simulink model "newPVmethod_1"  (R2024b)
settings: Solver=FixedStepDiscrete  StartTime=0.0  StopTime=20  FixedStep=1e-6  MaxStep=1e-6  MinStep=1e-6  RelTol=1e-3
values from neighbouring files (symbols this model uses):
  a0_ipv = kp_ipv*(1 + ts/ti_ipv)    (= 0.108333333333)    [PV_sim_init.m]    (also in controller_init.m = 0.0541666666667)
  a0_vpv = kp_vpv*(1 + ts/ti_vpv)    (= 0.100769230769)    [PV_sim_init.m]    (also in controller_init.m)
  a1_ipv = -kp_ipv    (= -0.1)    [PV_sim_init.m]    (also in controller_init.m = -0.05)
  a1_vpv = -kp_vpv    (= -0.1)    [PV_sim_init.m]    (also in controller_init.m)
  Vdc_sim = 400    [PV_sim_init.m]
undefined symbols (not defined in the file or in its folder): sigbuilder_block
libraries: spsSeriesRLCBranchLib x7, slpidlib x6, simulink x5, spsCurrentMeasurementLib x2, spsDCVoltageSourceLib x2, spsPVArrayLib x2, spsVoltageMeasurementLib x2, spsIGBTDiodeLib x2, spsControlledCurrentSourceLib x1, spsControlledVoltageSourceLib x1, spspowerguiLib x1, spsDiodeLib x1
(part 2 of 3)

== matlab function newPVmethod_1/basic_prc_2 ==
  data: Preserve input; c input; Vpv input; Ipv input; Vref output; timer input; D output; out output; reset input
function [Vref,D,out] = RefGen(Preserve,c,Vpv,Ipv,timer,reset)
% main function to execute every time

%variables to remember each execution
persistent state outprev
% global mppt_len measure_len operate_len MPP_SLOPE RESPOW_THRESH REPEAT_THRESH
% global NEW_POINT DEAD_CYCLES MAX_CYCLES

% mppt_len = 1;
% measure_len = 1;
% operate_len = 7;
MAX_CYCLES = 1999;
DEAD_CYCLES = MAX_CYCLES - 1000;
VREF_MAX = 360;
VREF_MIN = 0;
V_BUS_NOMINAL = 400;

%initialize
if isempty(state)
    state = init_state();
    state.Preserve = Preserve;
    outprev = zeros(1,2);
end
out = outprev;
Vref = state.Vrefprev;
dP = 0;
dV = 0;

% if Preserve == 100
%     % for i = 1:1:state.k
%     %     state.Ppva(i) = 0;
%     %     state.Vpva(i) = 0;
%     % end
%     % state.k = 1;
%     state.mode = 0;
%     % state.Preserve = Preserve;
% end

if c>DEAD_CYCLES && c<=MAX_CYCLES
    idx = c-DEAD_CYCLES;
    state.sampleVpv(idx) = Vpv;
    state.sampleIpv(idx) = Ipv;
    if c ~= MAX_CYCLES, state.f2 = 0; end  %f2 is used because there are 10 clock cycles per count of c
end
if c == MAX_CYCLES && ~state.f2 %calculate sample
    Vpv = mean(state.sampleVpv);
    Ppv = mean(state.sampleVpv.*state.sampleIpv);
    dV  = Vpv   - state.Vprev;
    dP  = Ppv - state.Pprev;
    if dP
        % state.mode = 0;
    switch state.mode
    case 0
        [Vref, state,out] = mppt_mode(state, Vpv, Ppv, dV, dP);
    case 1
        [Vref, state,out] = prc_measure_mode(state, Vpv, Ppv,dV,dP);
    case 2
        [Vref, state] = prc_operate_mode(state, Vpv, Ppv);
    end
    end
    state.Vprev = Vpv;
    state.Pprev = Ppv;
    state.f2 = 1;
    state.modeprev = state.mode;
end

out(1) = state.mode;
% out(2:4) = [state.Pp1m, state.Pp2m, state.Pp3m];
% out(5:7) = [state.Vp1m, state.Vp2m, state.Vp3m];
% out(8) = dP;
out(2) = state.k;
% out(10) = dV;
% use Vref result
if Vref >= VREF_MAX || Vref <= VREF_MIN
    Vref = state.Vrefprev;
end
D = 1 - Vref / V_BUS_NOMINAL;
state.Vrefprev = Vref;
outprev = out;
end

function s = init_state()

%INIT_STATE  Build a clean state struct for first-run initialisation.

s.sampleVpv  = zeros(1, 1000);
s.sampleIpv  = zeros(1, 1000);
s.Vprev      = 0;
s.Pprev      = 0;
s.Vrefprev   = 290;

% Mode: 0=MPPT, 1=PRC Measure, 2=PRC Operate
s.mode       = 0;
s.modeprev   = 0;

% MPPT / PRC shared
s.deltaVref  = 2;     % P&O perturbation step (V)
s.deltaVprc  = 1;     % PRC seek step (V)
s.Pmax       = 0;     % MPP power recorded at Mode-0 exit
s.Vmpp       = 0;     % MPP voltage recorded at Mode-0 exit
s.CVf        = 0;     % CV cold-start flag (set once per Mode-0 entry)
s.dir   = 1;     % MPPT direction
s.MPPf       = 0;

% Sub-optimal point storage (sorted, descending power)
s.Vpva       = zeros(1, 100);
s.Ppva       = zeros(1, 100);
s.k          = 1;     % next free slot in Vpva/Ppva
s.meas_succ = 0;
s.sortFail  = 0;
s.failCount = 0;
s.Vp1m = 0;  s.Pp1m = 0;
s.Vp2m = 0;  s.Pp2m = 0;
s.Vp3m = 0;  s.Pp3m = 0;


% Two-sample averaging temporaries
s.Vpvs       = zeros(1, 2);
s.Ppvs       = zeros(1, 2);
s.Vpvm       = 0;
s.Ppvm       = 0;

% Previous sub-optimal point (duplicate-rejection)
s.Vpvmpre    = 0;
s.Ppvmpre    = 0;

% sub-state flags
s.standby = 0;
s.standby2 = 0;
s.curve = 1;
s.f1 = 0;
s.f2 = 0;
s.f4 = 0;

% Quadratic fit coefficients (Mode 2)
s.A = 0;
s.B = 0;
s.C = 0;
s.Pcurve = 0;

s.numprc = 0;

end % init_state

%%%%%%%%%%%%%%%%%%%%%%%%%%%%%%%%%%
% ---- MPPT MODE 0 MAIN ----
%%%%%%%%%%%%%%%%%%%%%%%%%%%%%%%%%%
function [Vref,state,out] = mppt_mode(state,Vpv,Ppv,dV,dP)
MPP_SLOPE = 5;
out = zeros(1,2);

%re-initialize to create the jump
if state.MPPf
    Vref = state.Vmpp;
    state.MPPf = 0;
    return;
else
    Vref = state.Vrefprev;
end
if state.Pprev == 0             % on first execution
    return;
end

% typical P&0 logic using direction state
% direction init = 1
if Ppv > state.Pprev             
    if state.dir
        Vref = state.Vrefprev + state.deltaVref;
    else
        Vref = state.Vrefprev - state.deltaVref;
    end
else
    if state.dir
        Vref = state.Vrefprev - state.deltaVref;
        state.dir = 0;
    else
        Vref = state.Vrefprev + state.deltaVref;
        state.dir = 1;
    end
end
% check for max power with slope of PV curve
PVslope = abs(dP/dV);
if PVslope < MPP_SLOPE
    state.Pmax = Ppv;
    state.Vmpp  = Vpv;
    state.MPPf = 1;
    state.mode = 1;
    if Ppv < state.Preserve * 2.2  %low irradiance
        state.MPPf = 0;
        state.mode = 0;
    end
end
% out(8) = PVslope;
end

%%%%%%%%%%%%%%%%%%%%%%%%%%%%%%%%%%
% ---- MEASURE MODE 1 MAIN ----
%%%%%%%%%%%%%%%%%%%%%%%%%%%%%%%%%%
function [Vref, state, out] = prc_measure_mode(state, Vpv, Ppv,dV,dP)
REPEAT_THRESH_P = 30;
%REPEAT_THRESH_V = 0.01;
dV_THRESH = 0.05;
dP_THRESH = 1;
RESAMPLE_THRESH = 45;
RP_THRESH = 5;
out = zeros(1,2);
Vref = state.Vrefprev;
%Vref = state.Vrefprev;
if state.Vpvmpre && ~state.standby %jump to last known prc point
    Vref = state.Vpvmpre;
    state.Vpvmpre = 0;
    return;
end

%instead of these two, could try checking change in vref versus chang ein
%power
sameDir = (dV > dV_THRESH && dP >= -dP_THRESH) || (dV < -dV_THRESH && dP <= dP_THRESH);
notPmax = abs(state.Pmax - Ppv)/state.Preserve > 0.25;
if (Ppv < state.Preserve*1.1) %|| (sameDir && notPmax)
    state.Vpvmpre = 0;
    state.standby = 0;
    state.mode = 0;
    return;
end



if abs(Ppv - state.Ppvmpre) > RESAMPLE_THRESH
    state.standby2 = 0;
end

target = state.Pmax - state.Preserve;

% step towards target

state = updateDeltaVprc(state,Ppv);
if Vpv < state.Vmpp
    Vref = 1.05*(state.Vmpp);
    return;
else
    Vref = state.Vrefprev + state.deltaVprc;
% elseif Ppv > target
%     Vref = state.Vrefprev + state.deltaVprc;
% elseif Ppv < target
%     Vref = state.Vrefprev - state.deltaVprc;
end
state.numprc = state.numprc + 1;
if state.numprc >= 60
    state.Vpvmpre = Vpv;
    state.mode = 0;
    state.numprc = 0;
end

% check point validity
% onTarget = abs(Ppv - target) <= RP_THRESH;
% noRepeatP = min(abs(Ppv - state.Ppva)) >= REPEAT_THRESH_P;  %% change this to check the last 
% %noRepeatV = min(abs(Vpv - state.Vpva)) >= REPEAT_THRESH_V;
% if state.f4 == 1 && onTarget && ~state.standby %%fine search, close enough to check target
%     state.Vpvmpre = Vpv;
%     state.standby = 1;
%     rightSide = Vpv > state.Vmpp;
%     if(onTarget && rightSide && noRepeatP)% && noRepeatV)
%         [state,idxR] = insertPoint(state,Vpv,Ppv);
%         if state.k >= 4 && ~state.sortFail
%             state.mode = 2;
%             state.standby = 0;
%             state.standby2 = 0;
%             %state.failCount = 0;
%         elseif state.sortFail
%             %%state.failCount = state.failCount+1;
%             for i = idxR:1:state.k-1
%                 state.Vpva(i) = state.Vpva(i+1);
%                 state.Ppva(i) = state.Ppva(i+1);
%             end
%             state.k = state.k-1;
%             % state.Vpva = zeros(1,100);
%             % state.Ppva = zeros(1,100);
%             % state.k = 1;
%             state.sortFail = 0;
%             state.mode = 0;
%             state.standby = 0;
%             state.standby2 = 0;
%             %%state.failCount = 0;
%         end
%     end
%     state.f4 = 0;
% end
% % - close to Preserve?
% % - right side of PV curve
% % - far from other points?
% 
% if state.standby && ~state.standby2 && state.k >=4 && (Ppv > state.Ppva(state.k-1) && Ppv < state.Ppva(1))
%     state.mode = 2;
%     state.standby = 0;
%     state.standby2 = 0;
% elseif state.standby && noRepeatP && ~state.standby2
%     state.mode = 0;
%     state.standby = 0;
%     state.standby2 = 1;
%     state.Ppvmpre = Ppv;
% end


%semi-works%elseif state.standby && state.k >=4 && Ppv > state.Ppva(state.k-2)% || Ppv < state.Ppva(2))
end
%---------------

% MODE 1 HELPER 1
function s = updateDeltaVprc(s, Ppv) %for now, can re-tune or replace with controller
% Adaptive step size: coarse when far from target, fine when close.
    err = Ppv - abs(s.Pmax - s.Preserve);
    if err/(s.Pmax - s.Preserve) <= 0.025
        s.f4 = 1;
    end
    % 
    Kp = 1/34;
    Ki = 0;
    % s.errInt = s.errInt + err;
    s.deltaVprc = err*Kp;% + s.errInt*Ki;
    % if ~s.f1
    %     s.deltaVprc = Kp*err + Ki*s.errInt;
    % end

    %HIGH POWER LOOKUP TABLE
    % if     err >= 10000 && s.f1 == 0,  s.deltaVprc = 15;
    % elseif err >= 5000 && s.f1 == 0,  s.deltaVprc = 5;
    % elseif err >= 2000 && s.f1 == 0,  s.deltaVprc = 1.5;
    % elseif err >= 1000 && s.f1 == 0,  s.deltaVprc = 0.5;
    % elseif err >= 500  && s.f1 == 0,  s.deltaVprc = 0.25;
    % elseif err <= 300  && s.f1 == 0
    %     s.deltaVprc = 0.1;
    %     s.f4 = 1;           % fine enough to enable sampling
    % end
    % if     err >= 1000 && s.f1 == 0,  s.deltaVprc = 15;% + 0.0005*err;
    % elseif err >= 500 && s.f1 == 0,  s.deltaVprc = 10;
    % elseif err >= 200 && s.f1 == 0,  s.deltaVprc = 5;
    % elseif err >= 100 && s.f1 == 0,  s.deltaVprc = 2.5;
    % elseif err >= 50  && s.f1 == 0,  s.deltaVprc = 1;
    % elseif err <= 30  && s.f1 == 0
    %     s.deltaVprc = 0.25;
    %     s.f4 = 1;           % fine enough to enable sampling
    % end

    if s.standby == 1
        s.deltaVprc = 0;    % locked on target: hold position
    end
end

% MODE 1 HELPER 2
function [state,idxR] = insertPoint(state,Vpv,Ppv)
% find the new index the Ppv should be in
% check if the arrays w/ those new indices will be valid
% implement or return
idxV = state.k;
idxP = state.k;
idxR = 0;
for i = 1:state.k
    if Ppv > state.Ppva(i) %should be descending
        idxP = i;
        break;
    end
end
for i = 1:state.k
    if Vpv < state.Vpva(i) %should be ascending, init. to first 0 idx
        idxV = i;
        break;
    end
end

% violates curve shape requirement
if idxP ~= idxV
    state.sortFail = 1;
    idxR = idxV;
    return;
end

if state.k > 1
    for i = (state.k-1):-1:idxP  %shift the array to make room for new point
        state.Ppva(i+1) = state.Ppva(i);
        state.Vpva(i+1) = state.Vpva(i);
    end
end

%insert
state.Ppva(idxP) = Ppv;
state.Vpva(idxV) = Vpv;
state.k = state.k+1;
state.sortFail = 0;
end

%%%%%%%%%%%%%%%%%%%%%%%%%%%%%%%%%%
% ---- OPERATE MODE 2 MAIN ----
%%%%%%%%%%%%%%%%%%%%%%%%%%%%%%%%%%
function [Vref,s] = prc_operate_mode(s, Vpv, Ppv)

NEW_POINT = 100;
if Ppv > s.Ppva(2) || s.k == 3
    % Above second element: use the top three
    idx = [1, 2, 3];

elseif Ppv < s.Ppva(s.k-2)
    % Below second-to-last: use the bottom three
    idx = [s.k-3, s.k-2, s.k-1];

else
    % Linear scan for the bracketing pair
    % idx = [2, 3, 4];        % fallback
    minIdx = 2;
    minDiff = abs(Ppv-s.Ppva(minIdx));
    for i = 2:s.k-2 %og is k-3
        if abs(Ppv - s.Ppva(i)) < minDiff
            minDiff = abs(Ppv - s.Ppva(i));
            minIdx = i;
        end
        % if (Ppv - s.Ppva(i)) * (Ppv - s.Ppva(i+1)) < 0
        %     if abs(Ppv - s.Ppva(i)) >= abs(Ppv - s.Ppva(i+1))
        %         idx = [i,   i+1, i+2];
        %     else
        %         idx = [i-1, i,   i+1];
        %     end
        %     break;
        % end
    end
    idx = [minIdx-1, minIdx, minIdx+1];
end

%assign bracket points and do curve fitting

% s.Vp1m = s.Vpva(idx(1));  s.Pp1m = s.Ppva(idx(1));
% s.Vp2m = s.Vpva(idx(2));  s.Pp2m = s.Ppva(idx(2));
% s.Vp3m = s.Vpva(idx(3));  s.Pp3m = s.Ppva(idx(3));

% regression method
x = sum(s.Vpva);
x2 = sum(s.Vpva.^2);
x3 = sum(s.Vpva.^3);
x4 = sum(s.Vpva.^4);
y = sum(s.Ppva);
xy = sum(s.Vpva.*s.Ppva);
x2y = sum((s.Vpva.^2).*s.Ppva);
n = length(s.Vpva);

tmpA = [x4 x3 x2;
        x3 x2 x;
        x2 x  n;];
tmp_b = [x2y;xy;y;];
tmp_x = tmpA\tmp_b;

s.A  = tmp_x(1);
s.B  = tmp_x(2);
s.C  = tmp_x(3);
% % MATRIX METHOD
% tmpA = [s.Vp1m^2 s.Vp1m 1;
%         s.Vp2m^2 s.Vp2m 1;
%         s.Vp3m^2 s.Vp3m 1;];
% tmp_b = [s.Pp1m;s.Pp2m;s.Pp3m;];
% tmp_x = tmpA\tmp_b;
% 
% s.A  = tmp_x(1);
% s.B  = tmp_x(2);
% s.C  = tmp_x(3);

%SUBSTIUTION FORMULA
% dV21 = s.Vp2m - s.Vp1m;
% dV32 = s.Vp3m - s.Vp2m;
% dV13 = s.Vp1m - s.Vp3m;
% dP21 = s.Pp2m - s.Pp1m;
% dP32 = s.Pp3m - s.Pp2m;
% s.A  = (dP21*dV32 - dP32*dV21) / (dV21 * dV32 * dV13);
% s.B  = (dP21 - s.A*(s.Vp2m^2 - s.Vp1m^2)) / dV21;
% s.C  = s.Pp1m - s.A*s.Vp1m^2 - s.B*s.Vp1m;

s.Pcurve = s.A*Vpv^2 + s.B*Vpv + s.C;

Vcrit = -s.B/(2*s.A);
Pcrit = s.A*Vcrit^2 + s.B*Vcrit + s.C;

fallOff = (s.A < 0 && Ppv > Pcrit) || (s.A > 0 && Ppv < Pcrit); %promising, passed the short sim

% allRight = s.Vp1m > Vcrit;
% allLeft =  s.Vp3m < Vcrit; %conditions to find if the samples straddle critical point
% if ~(allRight || allLeft) %attempted fix
%     s.mode = 0;
%     s.standby = 1;
%     Vref = s.Vrefprev;
%     return;
% end
% if ~(allRight || allLeft) %attempted fix
%     idxR = s.k; 
% 
%     if s.Vp3m > Vcrit && s.Vp2m < Vcrit      %pick a point to remove based on 3 scenarios of straddling Vcrit
%         idxR = idx(3);
%     elseif s.Vp1m < Vcrit && s.Vp2m > Vcrit
%         idxR = idx(1);
%     elseif s.Vp2m == Vcrit
%         idxR = idx(2);
%     end
% 
%     for i = idxR:1:s.k-1
%     s.Vpva(i) = s.Vpva(i+1);
%     s.Ppva(i) = s.Ppva(i+1);
%     end
%     s.k = s.k-1;
% end


%wrongD =% (s.dir && Ppv > s.Pprev) || (~s.dir && Ppv < s.Pprev);  

% remove point opposite of critical point
% choose different selection


%diagnostic variables
%out(1) = s.Pcurve;
%step towards curve
if Ppv <= s.Pcurve
    Vref = s.Vrefprev + 0.25;
else
    Vref = s.Vrefprev - 0.25;
end

% fallOff = (s.Vrefprev <= Vcrit && Vcrit < Vref) || (s.Vrefprev > Vcrit && Vcrit >= Vref);
% if ~oneSide % just added, last stable point is vulnerable to this condition
%     [minP,idxV] = min(abs(s.Vpva - Vcrit));
%     for i = idxV:1:s.k-1
%         s.Vpva(i) = s.Vpva(i+1);
%         s.Ppva(i) = s.Ppva(i+1);
%     end
%     s.k = s.k-1;
%     s.mode = 0;
% end
lowIrr = Ppv < s.Preserve*1.1;
%check for stepping outside bracket range or falling off curve
if min(abs(Ppv - s.Ppva)) >= NEW_POINT || fallOff|| lowIrr || s.k < 4%abs(s.dir) >= 3 %wrongD %~oneSide || fallOff
    s.Vpvmpre = Vpv;
    s.mode = 0; %go get a new point
    s.standby2 = 0; %need a new point before we come back here
end
%check for low irradiance
end

== matlab function newPVmethod_1/stew_rewrite_left ==
  data: Preserve input; c input; Vpv input; Ipv input; Vref output; timer input; D output; out output; reset input
function [Vref,D,out] = RefGen(Preserve,c,Vpv,Ipv,timer,reset)
% main function to execute every time

%variables to remember each execution
persistent state outprev
% global mppt_len measure_len operate_len MPP_SLOPE RESPOW_THRESH REPEAT_THRESH
% global NEW_POINT DEAD_CYCLES MAX_CYCLES

% mppt_len = 1;
% measure_len = 1;
% operate_len = 7;
MAX_CYCLES = 399*5;
DEAD_CYCLES = MAX_CYCLES - 200;
VREF_MAX = 350;
VREF_MIN = 0;
V_BUS_NOMINAL = 400;

%initialize
if isempty(state)
    state = init_state();
    state.Preserve = Preserve;
    outprev = zeros(1,10);
end
out = outprev;
Vref = state.Vrefprev;
dP = 0;
dV = 0;
% if timer == 14.2
%     state.Preserve = Preserve;
% end
% if timer == TIMER_PERIOD || reset == 1
%         state = resetPRC(state);
% end
%sample for half cycle

if c>DEAD_CYCLES && c<=MAX_CYCLES
    idx = c-DEAD_CYCLES;
    state.sampleVpv(idx) = Vpv;
    state.sampleIpv(idx) = Ipv;
    if c ~= MAX_CYCLES, state.f2 = 0; end  %f2 is used because there are 10 clock cycles per count of c
end
if c == MAX_CYCLES && ~state.f2 %calculate sample
    Vpv = mean(state.sampleVpv);
    Ppv = mean(state.sampleVpv.*state.sampleIpv);
    dV  = Vpv   - state.Vprev;
    dP  = Ppv - state.Pprev;
    if dP
        % state.mode = 0;
    switch state.mode
    case 0
        [Vref, state,out] = mppt_mode(state, Vpv, Ppv, dV, dP);
    case 1
        [Vref, state,out] = prc_measure_mode(state, Vpv, Ppv,dV,dP);
    case 2
        [Vref, state] = prc_operate_mode(state, Vpv, Ppv);
    end
    end
    state.Vprev = Vpv;
    state.Pprev = Ppv;
    state.f2 = 1;
    state.modeprev = state.mode;
end

out(1) = state.mode;
out(2:4) = [state.Pp1m, state.Pp2m, state.Pp3m];
out(5:7) = [state.Vp1m, state.Vp2m, state.Vp3m];
out(8) = dP;
out(9) = state.k;
out(10) = dV;
% use Vref result
if Vref >= VREF_MAX || Vref <= VREF_MIN
    Vref = state.Vrefprev;
end
D = 1 - Vref / V_BUS_NOMINAL;
state.Vrefprev = Vref;
outprev = out;
end

function s = init_state()

%INIT_STATE  Build a clean state struct for first-run initialisation.

s.sampleVpv  = zeros(1, 200);
s.sampleIpv  = zeros(1, 200);
s.Vprev      = 0;
s.Pprev      = 0;
s.Vrefprev   = 290;

% Mode: 0=MPPT, 1=PRC Measure, 2=PRC Operate
s.mode       = 0;
s.modeprev   = 0;

% MPPT / PRC shared
s.deltaVref  = 1.5;     % P&O perturbation step (V)
s.deltaVprc  = 1;     % PRC seek step (V)
s.Pmax       = 0;     % MPP power recorded at Mode-0 exit
s.Vmpp       = 0;     % MPP voltage recorded at Mode-0 exit
s.CVf        = 0;     % CV cold-start flag (set once per Mode-0 entry)
s.dir   = 1;     % MPPT direction
s.MPPf       = 0;
s.errInt = 0;

% Sub-optimal point storage (sorted, descending power)
s.Vpva       = zeros(1, 100);
s.Ppva       = zeros(1, 100);
s.k          = 1;     % next free slot in Vpva/Ppva
s.meas_succ = 0;
s.sortFail  = 0;
s.failCount = 0;
s.Vp1m = 0;  s.Pp1m = 0;
s.Vp2m = 0;  s.Pp2m = 0;
s.Vp3m = 0;  s.Pp3m = 0;


% Two-sample averaging temporaries
s.Vpvs       = zeros(1, 2);
s.Ppvs       = zeros(1, 2);
s.Vpvm       = 0;
s.Ppvm       = 0;

% Previous sub-optimal point (duplicate-rejection)
s.Vpvmpre    = 0;
s.Ppvmpre    = 0;

% sub-state flags
s.standby = 0;
s.standby2 = 0;
s.curve = 1;
s.f1 = 0;
s.f2 = 0;
s.f4 = 0;

% Quadratic fit coefficients (Mode 2)
s.A = 0;
s.B = 0;
s.C = 0;
s.Pcurve = 0;

end % init_state

%%%%%%%%%%%%%%%%%%%%%%%%%%%%%%%%%%
% ---- MPPT MODE 0 MAIN ----
%%%%%%%%%%%%%%%%%%%%%%%%%%%%%%%%%%
function [Vref,state,out] = mppt_mode(state,Vpv,Ppv,dV,dP)
MPP_SLOPE = 5;
out = zeros(1,10);

%re-initialize to create the jump
if state.MPPf
    Vref = state.Vmpp;
    state.MPPf = 0;
    return;
else
    Vref = state.Vrefprev;
end
if state.Pprev == 0             % on first execution
    return;
end

% typical P&0 logic using direction state
% direction init = 1
if Ppv > state.Pprev             
    if state.dir
        Vref = state.Vrefprev + state.deltaVref;
    else
        Vref = state.Vrefprev - state.deltaVref;
    end
else
    if state.dir
        Vref = state.Vrefprev - state.deltaVref;
        state.dir = 0;
    else
        Vref = state.Vrefprev + state.deltaVref;
        state.dir = 1;
    end
end
% check for max power with slope of PV curve
PVslope = abs(dP/dV);
if PVslope < MPP_SLOPE
    state.Pmax = Ppv;
    state.Vmpp  = Vpv;
    state.MPPf = 1;
    state.mode = 1;
    if Ppv < state.Preserve * 2.2  %low irradiance
        state.MPPf = 0;
        state.mode = 0;
    end
end
out(8) = PVslope;
end

%%%%%%%%%%%%%%%%%%%%%%%%%%%%%%%%%%
% ---- MEASURE MODE 1 MAIN ----
%%%%%%%%%%%%%%%%%%%%%%%%%%%%%%%%%%
function [Vref, state, out] = prc_measure_mode(state, Vpv, Ppv,dV,dP)
REPEAT_THRESH_P = 60;
%REPEAT_THRESH_V = 0.01;
dV_THRESH = 0.05;
dP_THRESH = 1;
RESAMPLE_THRESH = 50;
RP_THRESH = 5;
out = zeros(1,10);
Vref = state.Vrefprev;
%Vref = state.Vrefprev;
% if state.Vpvmpre && ~state.standby %jump to last known prc point
%     Vref = state.Vpvmpre;
%     state.Vpvmpre = 0;
%     return;
% end
% sameDir = (dV > dV_THRESH && dP >= -dP_THRESH) || (dV < -dV_THRESH && dP <= dP_THRESH);
% notPmax = abs(state.Pmax - Ppv)/state.Preserve > 0.25;
if (Ppv < state.Preserve*1.1) %|| (sameDir && notPmax)
    state.Vpvmpre = 0;
    state.standby = 0;
    state.mode = 0;
    return;
end



if abs(Ppv - state.Ppvmpre) > RESAMPLE_THRESH
    state.standby2 = 0;
end

target = state.Pmax - state.Preserve;

% step towards target

state = updateDeltaVprc(state,Ppv);
if Vpv > state.Vmpp
    Vref = 0.95*(state.Vmpp);
    return;
else
    Vref = state.Vrefprev + state.deltaVprc;
% elseif Ppv > target
%     Vref = state.Vrefprev - state.deltaVprc;
% elseif Ppv < target
%     Vref = state.Vrefprev + state.deltaVprc;
end

% check point validity
onTarget = abs(Ppv - target) <= RP_THRESH;
noRepeatP = min(abs(Ppv - state.Ppva)) >= REPEAT_THRESH_P;  %% change this to check the last 
%noRepeatV = min(abs(Vpv - state.Vpva)) >= REPEAT_THRESH_V;
if state.f4 == 1 && onTarget && ~state.standby %%fine search, close enough to check target
    state.Vpvmpre = Vpv;
    state.standby = 1;
    rightSide = Vpv < state.Vmpp;
    if(onTarget && rightSide && noRepeatP)% && noRepeatV)
        [state,idxR] = insertPoint(state,Vpv,Ppv);
        if state.k >= 4 && ~state.sortFail
            state.mode = 2;
            state.standby = 0;
            state.standby2 = 0;
            %state.failCount = 0;
        elseif state.sortFail
            %%state.failCount = state.failCount+1;
            for i = idxR:1:state.k-1
                state.Vpva(i) = state.Vpva(i+1);
                state.Ppva(i) = state.Ppva(i+1);
            end
            state.k = state.k-1;
            % state.Vpva = zeros(1,100);
            % state.Ppva = zeros(1,100);
            % state.k = 1;
            state.sortFail = 0;
            state.mode = 0;
            state.standby = 0;
            state.standby2 = 0;
            %%state.failCount = 0;
        end
    end
    state.f4 = 0;
end
% - close to Preserve?
% - right side of PV curve
% - far from other points?

% add a standby that holds the Vref until a new point 

if state.standby && ~state.standby2 && state.k >=4 && (Ppv < state.Ppva(state.k-1) && Ppv > state.Ppva(1))
    state.mode = 2;
    state.standby = 0;
    state.standby2 = 0;
elseif state.standby && noRepeatP && ~state.standby2
    state.mode = 0;
    state.standby = 0;
    state.standby2 = 1;
    state.Ppvmpre = Ppv;
end


%semi-works%elseif state.standby && state.k >=4 && Ppv > state.Ppva(state.k-2)% || Ppv < state.Ppva(2))
end
%---------------

% MODE 1 HELPER 1
function s = updateDeltaVprc(s, Ppv) %for now, can re-tune or replace with controller
% Adaptive step size: coarse when far from target, fine when close.
    % err = abs(Ppv - abs(s.Pmax - s.Preserve));
    err = abs(s.Pmax - s.Preserve) - Ppv;
    if err/(s.Pmax - s.Preserve) <= 0.01
        s.f4 = 1;
    end
    % 
    % Kp = 0.0001;
    % Ki = 0;
    s.errInt = s.errInt + err;
    % if ~s.f1
    %     s.deltaVprc = Kp*err + Ki*s.errInt;
    % end


    % if     err >= 1000 && s.f1 == 0,  s.deltaVprc = 15;% + 0.0005*err;
    % elseif err >= 500 && s.f1 == 0,  s.deltaVprc = 10;
    % elseif err >= 200 && s.f1 == 0,  s.deltaVprc = 5;
    % elseif err >= 100 && s.f1 == 0,  s.deltaVprc = 2.5;
    % elseif err >= 50  && s.f1 == 0,  s.deltaVprc = 1;
    % elseif err <= 30  && s.f1 == 0
    %     s.deltaVprc = 0.25;
    %     s.f4 = 1;           % fine enough to enable sampling
    % end
    Kp = 1/7.2; %34 is right side
    Ki = 0;
    s.deltaVprc = err*Kp + Ki*s.errInt;
    if s.standby == 1
        s.deltaVprc = 0;    % locked on target: hold position
    end
end

% MODE 1 HELPER 2
function [state,idxR] = insertPoint(state,Vpv,Ppv)
% find the new index the Ppv should be in
% check if the arrays w/ those new indices will be valid
% implement or return
idxV = state.k;
idxP = state.k;
idxR = 0;
for i = 1:state.k
    if Ppv < state.Ppva(i) %should be ascending
        idxP = i;
        break;
    end
end
for i = 1:state.k
    if Vpv < state.Vpva(i) %should be ascending, init. to first 0 idx
        idxV = i;
        break;
    end
end

% violates curve shape requirement
if idxP ~= idxV
    state.sortFail = 1;
    idxR = idxV;
    return;
end

if state.k > 1
    for i = (state.k-1):-1:idxP  %shift the array to make room for new point
        state.Ppva(i+1) = state.Ppva(i);
        state.Vpva(i+1) = state.Vpva(i);
    end
end

%insert
state.Ppva(idxP) = Ppv;
state.Vpva(idxV) = Vpv;
state.k = state.k+1;
state.sortFail = 0;
end

%%%%%%%%%%%%%%%%%%%%%%%%%%%%%%%%%%
% ---- OPERATE MODE 2 MAIN ----
%%%%%%%%%%%%%%%%%%%%%%%%%%%%%%%%%%
function [Vref,s] = prc_operate_mode(s, Vpv, Ppv)

NEW_POINT = 100;
if Ppv < s.Ppva(2) || s.k == 3
    % Above second element: use the top three
    idx = [1, 2, 3];

elseif Ppv > s.Ppva(s.k-2)
    % Below second-to-last: use the bottom three
    idx = [s.k-3, s.k-2, s.k-1];

else
    % Linear scan for the bracketing pair
    % idx = [2, 3, 4];        % fallback
    minIdx = 2;
    minDiff = abs(Ppv-s.Ppva(minIdx));
    for i = 2:s.k-2 %og is k-3
        if abs(Ppv - s.Ppva(i)) < minDiff
            minDiff = abs(Ppv - s.Ppva(i));
            minIdx = i;
        end
        % if (Ppv - s.Ppva(i)) * (Ppv - s.Ppva(i+1)) < 0
        %     if abs(Ppv - s.Ppva(i)) >= abs(Ppv - s.Ppva(i+1))
        %         idx = [i,   i+1, i+2];
        %     else
        %         idx = [i-1, i,   i+1];
        %     end
        %     break;
        % end
    end
    idx = [minIdx-1, minIdx, minIdx+1];
end

%assign bracket points and do curve fitting

s.Vp1m = s.Vpva(idx(1));  s.Pp1m = s.Ppva(idx(1));
s.Vp2m = s.Vpva(idx(2));  s.Pp2m = s.Ppva(idx(2));
s.Vp3m = s.Vpva(idx(3));  s.Pp3m = s.Ppva(idx(3));

% % MATRIX METHOD
% tmpA = [s.Vp1m^2 s.Vp1m 1;
%         s.Vp2m^2 s.Vp2m 1;
%         s.Vp3m^2 s.Vp3m 1;];
% tmp_b = [s.Pp1m;s.Pp2m;s.Pp3m;];
% tmp_x = tmpA\tmp_b;
% 
% s.A  = tmp_x(1);
% s.B  = tmp_x(2);
% s.C  = tmp_x(3);

%SUBSTIUTION FORMULA
dV21 = s.Vp2m - s.Vp1m;
dV32 = s.Vp3m - s.Vp2m;
dV13 = s.Vp1m - s.Vp3m;
dP21 = s.Pp2m - s.Pp1m;
dP32 = s.Pp3m - s.Pp2m;
s.A  = (dP21*dV32 - dP32*dV21) / (dV21 * dV32 * dV13);
s.B  = (dP21 - s.A*(s.Vp2m^2 - s.Vp1m^2)) / dV21;
s.C  = s.Pp1m - s.A*s.Vp1m^2 - s.B*s.Vp1m;

s.Pcurve = s.A*Vpv^2 + s.B*Vpv + s.C;

Vcrit = -s.B/(2*s.A);
Pcrit = s.A*Vcrit^2 + s.B*Vcrit + s.C;

fallOff = (s.A < 0 && Ppv > Pcrit) || (s.A > 0 && Ppv < Pcrit); %promising, passed the short sim

% allRight = s.Vp1m > Vcrit;
% allLeft =  s.Vp3m < Vcrit; %conditions to find if the samples straddle critical point
% if ~(allRight || allLeft) %attempted fix
%     s.mode = 0;
%     s.standby = 1;
%     Vref = s.Vrefprev;
%     return;
% end
% if ~(allRight || allLeft) %attempted fix
%     idxR = s.k; 
% 
%     if s.Vp3m > Vcrit && s.Vp2m < Vcrit      %pick a point to remove based on 3 scenarios of straddling Vcrit
%         idxR = idx(3);
%     elseif s.Vp1m < Vcrit && s.Vp2m > Vcrit
%         idxR = idx(1);
%     elseif s.Vp2m == Vcrit
%         idxR = idx(2);
%     end
% 
%     for i = idxR:1:s.k-1
%     s.Vpva(i) = s.Vpva(i+1);
%     s.Ppva(i) = s.Ppva(i+1);
%     end
%     s.k = s.k-1;
% end


%wrongD =% (s.dir && Ppv > s.Pprev) || (~s.dir && Ppv < s.Pprev);  

% remove point opposite of critical point
% choose different selection


%diagnostic variables
%out(1) = s.Pcurve;
%step towards curve
if Ppv <= s.Pcurve
    Vref = s.Vrefprev - 0.25;
else
    Vref = s.Vrefprev + 0.25;
end

% fallOff = (s.Vrefprev <= Vcrit && Vcrit < Vref) || (s.Vrefprev > Vcrit && Vcrit >= Vref);
% if ~oneSide % just added, last stable point is vulnerable to this condition
%     [minP,idxV] = min(abs(s.Vpva - Vcrit));
%     for i = idxV:1:s.k-1
%         s.Vpva(i) = s.Vpva(i+1);
%         s.Ppva(i) = s.Ppva(i+1);
%     end
%     s.k = s.k-1;
%     s.mode = 0;
% end
lowIrr = Ppv < s.Preserve*1.1;
%check for stepping outside bracket range or falling off curve
if min(abs(Ppv - s.Ppva)) >= NEW_POINT|| fallOff || lowIrr || s.k < 4%abs(s.dir) >= 3 %wrongD %~oneSide || fallOff 
    s.Vpvmpre = Vpv;
    s.mode = 0; %go get a new point
    % s.standby2 = 0; %need a new point before we come back here
end
%check for low irradiance
end

== matlab function newPVmethod_1/switching model/vscode pi_ctrl ==
  data: ypre input; err input; errpre input; y output; a0 input; a1 input
function y = fcn(ypre,err,errpre,a0,a1)
max = 15;
min = -8;
temp = ypre + a0*err + a1*errpre;
if temp > max
    y = max;
elseif temp < min
    y = min;
else
    y = temp;
end

== matlab function newPVmethod_1/MPPT ==
  data: c input; Vref output; Vpv input; Ipv input; D output; P output; Vmpp output; test output
function [Vref,D,P,Vmpp,test]= RefGen(c,Vpv,Ipv)  %Vref is the mppt output and V,I are inputs

persistent MPPT_dir Vprev Pprev Vrefprev sampleIpv sampleVpv Ppv dP dV f2;
% Kp=0.001;
% Ki=1e-4;
% Ti=0.02;
if isempty(MPPT_dir)
    MPPT_dir = 1;
    Pprev = 0;
    Vprev = 0;
    Vrefprev = 250;
    sampleIpv = zeros(1,200);
    sampleVpv = zeros(1,200);
    Ppv = 0;
    dP = 0;
    dV = 0;
    f2 = 0;
end
deltaVref = 1;

DEAD_CYCLES = 199;
MAX_CYCLES = 399;
Vref = Vrefprev;
if c>DEAD_CYCLES && c<=MAX_CYCLES
    idx = c-DEAD_CYCLES;
    sampleVpv(idx) = Vpv;
    sampleIpv(idx) = Ipv;
    if c~= MAX_CYCLES, f2 = 0; end
end
if c == MAX_CYCLES && ~f2 %calculate sample
    Vpv = mean(sampleVpv);
    Ppv = mean(sampleVpv.*sampleIpv);
    dV  = Vpv   - Vprev;
    dP  = Ppv - Pprev;
    if dP && Pprev
    if Ppv > Pprev             
        if MPPT_dir
            Vref = Vrefprev + deltaVref;
        else
            Vref = Vrefprev - deltaVref;
        end
    else
        if MPPT_dir
            Vref = Vrefprev - deltaVref;
            MPPT_dir = 0;
        else
            Vref = Vrefprev + deltaVref;
            MPPT_dir = 1;
        end
    end
    end
    Vprev = Vpv;
    Pprev = Ppv;
    f2 = 1;
end
Vrefprev = Vref;
test = abs(dP/dV);
D = Vref/400;
P = Ppv;
Vmpp = Vpv;

end

== matlab function newPVmethod_1/switching model/vscode pi_ctrl1 ==
  data: ypre input; err input; errpre input; y output; a0 input; a1 input
function y = fcn(ypre,err,errpre,a0,a1)
max = 0.99;
min = 0.01;
temp = ypre + a0*err + a1*errpre;
if temp > max
    y = max;
elseif temp < min
    y = min;
else
    y = temp;
end

== matlab function newPVmethod_1/switching model/vscode pi_ctrl2 ==
  data: ypre input; err input; errpre input; y output; a0 input; a1 input
function y = fcn(ypre,err,errpre,a0,a1)

y = ypre + a0*err + a1*errpre;

== matlab function newPVmethod_1/switching model/vscode pi_ctrl3 ==
  data: ypre input; err input; errpre input; y output; a0 input; a1 input
function y = fcn(ypre,err,errpre,a0,a1)

y = ypre + a0*err + a1*errpre;

== matlab function newPVmethod_1/stew_regression ==
  data: Preserve input; c input; Vpv input; Ipv input; Vref output; timer input; D output; out output; reset input
function [Vref,D,out] = RefGen(Preserve,c,Vpv,Ipv,timer,reset)
% main function to execute every time

%variables to remember each execution
persistent state outprev
% global mppt_len measure_len operate_len MPP_SLOPE RESPOW_THRESH REPEAT_THRESH
% global NEW_POINT DEAD_CYCLES MAX_CYCLES

% mppt_len = 1;
% measure_len = 1;
% operate_len = 7;
MAX_CYCLES = 399;
DEAD_CYCLES = MAX_CYCLES - 200;
VREF_MAX = 360;
VREF_MIN = 0;
V_BUS_NOMINAL = 400;

%initialize
if isempty(state)
    state = init_state();
    state.Preserve = Preserve;
    outprev = zeros(1,2);
end
out = outprev;
Vref = state.Vrefprev;
dP = 0;
dV = 0;

% if Preserve == 100
%     % for i = 1:1:state.k
%     %     state.Ppva(i) = 0;
%     %     state.Vpva(i) = 0;
%     % end
%     % state.k = 1;
%     state.mode = 0;
%     % state.Preserve = Preserve;
% end

if c>DEAD_CYCLES && c<=MAX_CYCLES
    idx = c-DEAD_CYCLES;
    state.sampleVpv(idx) = Vpv;
    state.sampleIpv(idx) = Ipv;
    if c ~= MAX_CYCLES, state.f2 = 0; end  %f2 is used because there are 10 clock cycles per count of c
end
if c == MAX_CYCLES && ~state.f2 %calculate sample
    Vpv = mean(state.sampleVpv);
    Ppv = mean(state.sampleVpv.*state.sampleIpv);
    dV  = Vpv   - state.Vprev;
    dP  = Ppv - state.Pprev;
    if dP
        % state.mode = 0;
    switch state.mode
    case 0
        [Vref, state,out] = mppt_mode(state, Vpv, Ppv, dV, dP);
    case 1
        [Vref, state,out] = prc_measure_mode(state, Vpv, Ppv,dV,dP);
    case 2
        [Vref, state] = prc_operate_mode(state, Vpv, Ppv);
    end
    end
    state.Vprev = Vpv;
    state.Pprev = Ppv;
    state.f2 = 1;
    state.modeprev = state.mode;
end

out(1) = state.mode;
% out(2:4) = [state.Pp1m, state.Pp2m, state.Pp3m];
% out(5:7) = [state.Vp1m, state.Vp2m, state.Vp3m];
% out(8) = dP;
out(2) = state.k;
% out(10) = dV;
% use Vref result
if Vref >= VREF_MAX || Vref <= VREF_MIN
    Vref = state.Vrefprev;
end
D = 1 - Vref / V_BUS_NOMINAL;
state.Vrefprev = Vref;
outprev = out;
end

function s = init_state()

%INIT_STATE  Build a clean state struct for first-run initialisation.

s.sampleVpv  = zeros(1, 200);
s.sampleIpv  = zeros(1, 200);
s.Vprev      = 0;
s.Pprev      = 0;
s.Vrefprev   = 290;

% Mode: 0=MPPT, 1=PRC Measure, 2=PRC Operate
s.mode       = 0;
s.modeprev   = 0;

% MPPT / PRC shared
s.deltaVref  = 2;     % P&O perturbation step (V)
s.deltaVprc  = 1;     % PRC seek step (V)
s.Pmax       = 0;     % MPP power recorded at Mode-0 exit
s.Vmpp       = 0;     % MPP voltage recorded at Mode-0 exit
s.CVf        = 0;     % CV cold-start flag (set once per Mode-0 entry)
s.dir   = 1;     % MPPT direction
s.MPPf       = 0;

% Sub-optimal point storage (sorted, descending power)
s.Vpva       = zeros(1, 100);
s.Ppva       = zeros(1, 100);
s.k          = 1;     % next free slot in Vpva/Ppva
s.meas_succ = 0;
s.sortFail  = 0;
s.failCount = 0;
s.Vp1m = 0;  s.Pp1m = 0;
s.Vp2m = 0;  s.Pp2m = 0;
s.Vp3m = 0;  s.Pp3m = 0;


% Two-sample averaging temporaries
s.Vpvs       = zeros(1, 2);
s.Ppvs       = zeros(1, 2);
s.Vpvm       = 0;
s.Ppvm       = 0;

% Previous sub-optimal point (duplicate-rejection)
s.Vpvmpre    = 0;
s.Ppvmpre    = 0;

% sub-state flags
s.standby = 0;
s.standby2 = 0;
s.curve = 1;
s.f1 = 0;
s.f2 = 0;
s.f4 = 0;

% Quadratic fit coefficients (Mode 2)
s.A = 0;
s.B = 0;
s.C = 0;
s.Pcurve = 0;

end % init_state

%%%%%%%%%%%%%%%%%%%%%%%%%%%%%%%%%%
% ---- MPPT MODE 0 MAIN ----
%%%%%%%%%%%%%%%%%%%%%%%%%%%%%%%%%%
function [Vref,state,out] = mppt_mode(state,Vpv,Ppv,dV,dP)
MPP_SLOPE = 5;
out = zeros(1,2);

%re-initialize to create the jump
if state.MPPf
    Vref = state.Vmpp;
    state.MPPf = 0;
    return;
else
    Vref = state.Vrefprev;
end
if state.Pprev == 0             % on first execution
    return;
end

% typical P&0 logic using direction state
% direction init = 1
if Ppv > state.Pprev             
    if state.dir
        Vref = state.Vrefprev + state.deltaVref;
    else
        Vref = state.Vrefprev - state.deltaVref;
    end
else
    if state.dir
        Vref = state.Vrefprev - state.deltaVref;
        state.dir = 0;
    else
        Vref = state.Vrefprev + state.deltaVref;
        state.dir = 1;
    end
end
% check for max power with slope of PV curve
PVslope = abs(dP/dV);
if PVslope < MPP_SLOPE
    state.Pmax = Ppv;
    state.Vmpp  = Vpv;
    state.MPPf = 1;
    state.mode = 1;
    if Ppv < state.Preserve * 2.2  %low irradiance
        state.MPPf = 0;
        state.mode = 0;
    end
end
% out(8) = PVslope;
end

%%%%%%%%%%%%%%%%%%%%%%%%%%%%%%%%%%
% ---- MEASURE MODE 1 MAIN ----
%%%%%%%%%%%%%%%%%%%%%%%%%%%%%%%%%%
function [Vref, state, out] = prc_measure_mode(state, Vpv, Ppv,dV,dP)
REPEAT_THRESH_P = 30;
%REPEAT_THRESH_V = 0.01;
dV_THRESH = 0.05;
dP_THRESH = 1;
RESAMPLE_THRESH = 25;
RP_THRESH = 5;
out = zeros(1,2);
Vref = state.Vrefprev;
%Vref = state.Vrefprev;
if state.Vpvmpre && ~state.standby %jump to last known prc point
    Vref = state.Vpvmpre;
    state.Vpvmpre = 0;
    return;
end

%instead of these two, could try checking change in vref versus chang ein
%power
sameDir = (dV > dV_THRESH && dP >= -dP_THRESH) || (dV < -dV_THRESH && dP <= dP_THRESH);
notPmax = abs(state.Pmax - Ppv)/state.Preserve > 0.25;
if (Ppv < state.Preserve*1.1) || (sameDir && notPmax)
    state.Vpvmpre = 0;
    state.standby = 0;
    state.mode = 0;
    return;
end



if abs(Ppv - state.Ppvmpre) > REPEAT_THRESH_P
    state.standby2 = 0;
end

target = state.Pmax - state.Preserve;

% step towards target

state = updateDeltaVprc(state,Ppv);
if Vpv < state.Vmpp
    Vref = 1.05*(state.Vmpp);
    return;
else
    Vref = state.Vrefprev + state.deltaVprc;
% elseif Ppv > target
%     Vref = state.Vrefprev + state.deltaVprc;
% elseif Ppv < target
%     Vref = state.Vrefprev - state.deltaVprc;
end

% check point validity
onTarget = abs(Ppv - target) <= RP_THRESH;
noRepeatP = min(abs(Ppv - state.Ppva)) >= REPEAT_THRESH_P;  %% change this to check the last 
%noRepeatV = min(abs(Vpv - state.Vpva)) >= REPEAT_THRESH_V;
if state.f4 == 1 && onTarget && ~state.standby %%fine search, close enough to check target
    state.Vpvmpre = Vpv;
    state.standby = 1;
    rightSide = Vpv > state.Vmpp;
    if(onTarget && rightSide && noRepeatP)% && noRepeatV)
        [state,idxR] = insertPoint(state,Vpv,Ppv);
        if state.k >= 4 && ~state.sortFail
            state.mode = 2;
            state.standby = 0;
            state.standby2 = 0;
            %state.failCount = 0;
        elseif state.sortFail
            %%state.failCount = state.failCount+1;
            for i = idxR:1:state.k-1
                state.Vpva(i) = state.Vpva(i+1);
                state.Ppva(i) = state.Ppva(i+1);
            end
            state.k = state.k-1;
            % state.Vpva = zeros(1,100);
            % state.Ppva = zeros(1,100);
            % state.k = 1;
            state.sortFail = 0;
            state.mode = 0;
            state.standby = 0;
            state.standby2 = 0;
            %%state.failCount = 0;
        end
    end
    state.f4 = 0;
end
% - close to Preserve?
% - right side of PV curve
% - far from other points?

% add a standby that holds the Vref until a new point 

if state.standby && ~state.standby2 && state.k >=4 && (Ppv > state.Ppva(state.k-1) && Ppv < state.Ppva(1))
    state.mode = 2;
    state.standby = 0;
    state.standby2 = 0;
elseif state.standby && noRepeatP && ~state.standby2
    state.mode = 0;
    state.standby = 0;
    state.standby2 = 1;
    state.Ppvmpre = Ppv;
end


%semi-works%elseif state.standby && state.k >=4 && Ppv > state.Ppva(state.k-2)% || Ppv < state.Ppva(2))
end
%---------------

% MODE 1 HELPER 1
function s = updateDeltaVprc(s, Ppv) %for now, can re-tune or replace with controller
% Adaptive step size: coarse when far from target, fine when close.
    err = Ppv - abs(s.Pmax - s.Preserve);
    if err/(s.Pmax - s.Preserve) <= 0.025
        s.f4 = 1;
    end
    % 
    Kp = 1/34;
    Ki = 0;
    % s.errInt = s.errInt + err;
    s.deltaVprc = err*Kp;% + s.errInt*Ki;
    % if ~s.f1
    %     s.deltaVprc = Kp*err + Ki*s.errInt;
    % end

    %HIGH POWER LOOKUP TABLE
    % if     err >= 10000 && s.f1 == 0,  s.deltaVprc = 15;
    % elseif err >= 5000 && s.f1 == 0,  s.deltaVprc = 5;
    % elseif err >= 2000 && s.f1 == 0,  s.deltaVprc = 1.5;
    % elseif err >= 1000 && s.f1 == 0,  s.deltaVprc = 0.5;
    % elseif err >= 500  && s.f1 == 0,  s.deltaVprc = 0.25;
    % elseif err <= 300  && s.f1 == 0
    %     s.deltaVprc = 0.1;
    %     s.f4 = 1;           % fine enough to enable sampling
    % end
    % if     err >= 1000 && s.f1 == 0,  s.deltaVprc = 15;% + 0.0005*err;
    % elseif err >= 500 && s.f1 == 0,  s.deltaVprc = 10;
    % elseif err >= 200 && s.f1 == 0,  s.deltaVprc = 5;
    % elseif err >= 100 && s.f1 == 0,  s.deltaVprc = 2.5;
    % elseif err >= 50  && s.f1 == 0,  s.deltaVprc = 1;
    % elseif err <= 30  && s.f1 == 0
    %     s.deltaVprc = 0.25;
    %     s.f4 = 1;           % fine enough to enable sampling
    % end

    if s.standby == 1
        s.deltaVprc = 0;    % locked on target: hold position
    end
end

% MODE 1 HELPER 2
function [state,idxR] = insertPoint(state,Vpv,Ppv)
% find the new index the Ppv should be in
% check if the arrays w/ those new indices will be valid
% implement or return
idxV = state.k;
idxP = state.k;
idxR = 0;
% for i = 1:state.k
%     if Ppv > state.Ppva(i) %should be descending
%         idxP = i;
%         break;
%     end
% end
% for i = 1:state.k
%     if Vpv < state.Vpva(i) %should be ascending, init. to first 0 idx
%         idxV = i;
%         break;
%     end
% end
% 
% % violates curve shape requirement
% if idxP ~= idxV
%     state.sortFail = 1;
%     idxR = idxV;
%     return;
% end
% 
% if state.k > 1
%     for i = (state.k-1):-1:idxP  %shift the array to make room for new point
%         state.Ppva(i+1) = state.Ppva(i);
%         state.Vpva(i+1) = state.Vpva(i);
%     end
% end

%insert
state.Ppva(idxP) = Ppv;
state.Vpva(idxV) = Vpv;
state.k = state.k+1;
state.sortFail = 0;
end

%%%%%%%%%%%%%%%%%%%%%%%%%%%%%%%%%%
% ---- OPERATE MODE 2 MAIN ----
%%%%%%%%%%%%%%%%%%%%%%%%%%%%%%%%%%
function [Vref,s] = prc_operate_mode(s, Vpv, Ppv)

NEW_POINT = 100;
% if Ppv > s.Ppva(2) || s.k == 3
%     % Above second element: use the top three
%     idx = [1, 2, 3];
% 
% elseif Ppv < s.Ppva(s.k-2)
%     % Below second-to-last: use the bottom three
%     idx = [s.k-3, s.k-2, s.k-1];
% 
% else
%     % Linear scan for the bracketing pair
%     % idx = [2, 3, 4];        % fallback
%     minIdx = 2;
%     minDiff = abs(Ppv-s.Ppva(minIdx));
%     for i = 2:s.k-2 %og is k-3
%         if abs(Ppv - s.Ppva(i)) < minDiff
%             minDiff = abs(Ppv - s.Ppva(i));
%             minIdx = i;
%         end
%         % if (Ppv - s.Ppva(i)) * (Ppv - s.Ppva(i+1)) < 0
%         %     if abs(Ppv - s.Ppva(i)) >= abs(Ppv - s.Ppva(i+1))
%         %         idx = [i,   i+1, i+2];
%         %     else
%         %         idx = [i-1, i,   i+1];
%         %     end
%         %     break;
%         % end
%     end
%     idx = [minIdx-1, minIdx, minIdx+1];
% end

%assign bracket points and do curve fitting

% s.Vp1m = s.Vpva(idx(1));  s.Pp1m = s.Ppva(idx(1));
% s.Vp2m = s.Vpva(idx(2));  s.Pp2m = s.Ppva(idx(2));
% s.Vp3m = s.Vpva(idx(3));  s.Pp3m = s.Ppva(idx(3));

% regression method
x = sum(s.Vpva);
x2 = sum(s.Vpva.^2);
x3 = sum(s.Vpva.^3);
x4 = sum(s.Vpva.^4);
y = sum(s.Ppva);
xy = sum(s.Vpva.*s.Ppva);
x2y = sum((s.Vpva.^2).*s.Ppva);
n = length(s.Vpva);

tmpA = [x4 x3 x2;
        x3 x2 x;
        x2 x  n;];
tmp_b = [x2y;xy;y;];
tmp_x = tmpA\tmp_b;

s.A  = tmp_x(1);
s.B  = tmp_x(2);
s.C  = tmp_x(3);
% % MATRIX METHOD
% tmpA = [s.Vp1m^2 s.Vp1m 1;
%         s.Vp2m^2 s.Vp2m 1;
%         s.Vp3m^2 s.Vp3m 1;];
% tmp_b = [s.Pp1m;s.Pp2m;s.Pp3m;];
% tmp_x = tmpA\tmp_b;
% 
% s.A  = tmp_x(1);
% s.B  = tmp_x(2);
% s.C  = tmp_x(3);

%SUBSTIUTION FORMULA
% dV21 = s.Vp2m - s.Vp1m;
% dV32 = s.Vp3m - s.Vp2m;
% dV13 = s.Vp1m - s.Vp3m;
% dP21 = s.Pp2m - s.Pp1m;
% dP32 = s.Pp3m - s.Pp2m;
% s.A  = (dP21*dV32 - dP32*dV21) / (dV21 * dV32 * dV13);
% s.B  = (dP21 - s.A*(s.Vp2m^2 - s.Vp1m^2)) / dV21;
% s.C  = s.Pp1m - s.A*s.Vp1m^2 - s.B*s.Vp1m;

s.Pcurve = s.A*Vpv^2 + s.B*Vpv + s.C;

Vcrit = -s.B/(2*s.A);
Pcrit = s.A*Vcrit^2 + s.B*Vcrit + s.C;

fallOff = (s.A < 0 && Ppv > Pcrit) || (s.A > 0 && Ppv < Pcrit); %promising, passed the short sim

% allRight = s.Vp1m > Vcrit;
% allLeft =  s.Vp3m < Vcrit; %conditions to find if the samples straddle critical point
% if ~(allRight || allLeft) %attempted fix
%     s.mode = 0;
%     s.standby = 1;
%     Vref = s.Vrefprev;
%     return;
% end
% if ~(allRight || allLeft) %attempted fix
%     idxR = s.k; 
% 
%     if s.Vp3m > Vcrit && s.Vp2m < Vcrit      %pick a point to remove based on 3 scenarios of straddling Vcrit
%         idxR = idx(3);
%     elseif s.Vp1m < Vcrit && s.Vp2m > Vcrit
%         idxR = idx(1);
%     elseif s.Vp2m == Vcrit
%         idxR = idx(2);
%     end
% 
%     for i = idxR:1:s.k-1
%     s.Vpva(i) = s.Vpva(i+1);
%     s.Ppva(i) = s.Ppva(i+1);
%     end
%     s.k = s.k-1;
% end


%wrongD =% (s.dir && Ppv > s.Pprev) || (~s.dir && Ppv < s.Pprev);  

% remove point opposite of critical point
% choose different selection


%diagnostic variables
%out(1) = s.Pcurve;
%step towards curve
if Ppv <= s.Pcurve
    Vref = s.Vrefprev + 0.25;
else
    Vref = s.Vrefprev - 0.25;
end

% fallOff = (s.Vrefprev <= Vcrit && Vcrit < Vref) || (s.Vrefprev > Vcrit && Vcrit >= Vref);
% if ~oneSide % just added, last stable point is vulnerable to this condition
%     [minP,idxV] = min(abs(s.Vpva - Vcrit));
%     for i = idxV:1:s.k-1
%         s.Vpva(i) = s.Vpva(i+1);
%         s.Ppva(i) = s.Ppva(i+1);
%     end
%     s.k = s.k-1;
%     s.mode = 0;
% end
lowIrr = Ppv < s.Preserve*1.1;
%check for stepping outside bracket range or falling off curve
if min(abs(Ppv - s.Ppva)) >= NEW_POINT || fallOff|| lowIrr || s.k < 4%abs(s.dir) >= 3 %wrongD %~oneSide || fallOff
    s.Vpvmpre = Vpv;
    s.mode = 0; %go get a new point
    s.standby2 = 0; %need a new point before we come back here
end
%check for low irradiance
end
